simulink model "reference_frames_development"  (R2022a)
settings: Solver=VariableStepAuto  StartTime=0.0  StopTime=10.0  RelTol=1e-3
settings Model: Creator=samuel  LastModifiedBy=samuel

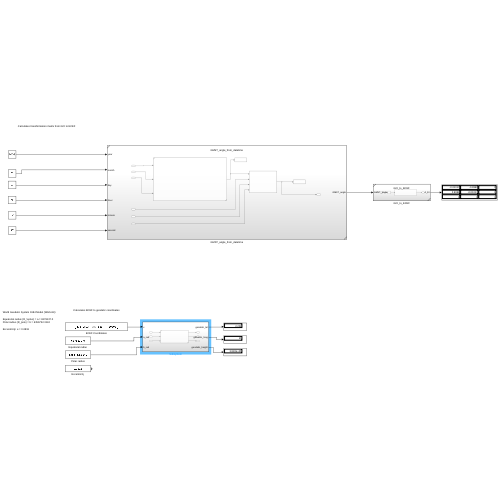
[thumbnail: Simulink's stored preview of the top-level diagram]
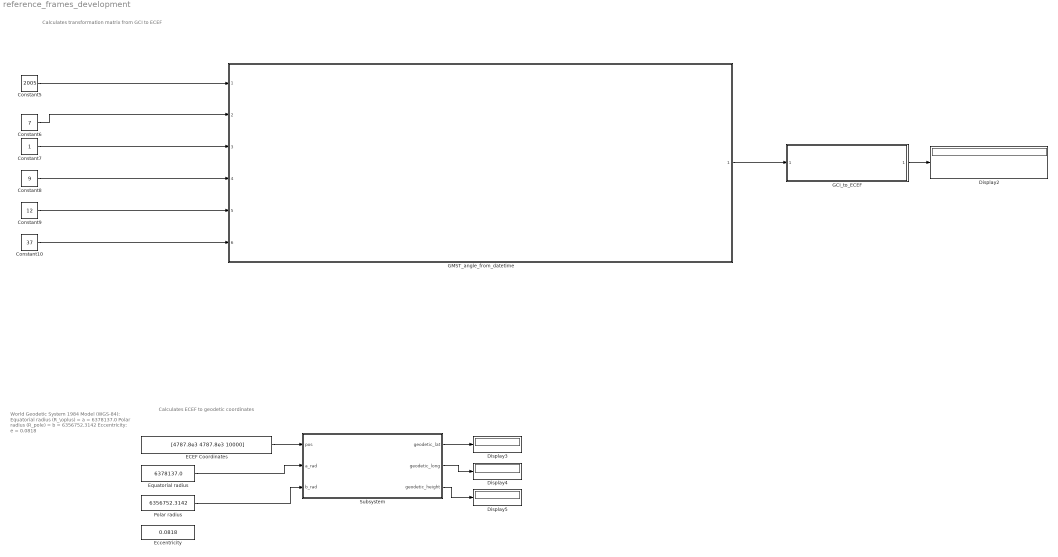
== system reference_frames_development ==
  note: Calculates transformation matrix from GCI to ECEF
  note: Calculates ECEF to geodetic coordinates
  note: World Geodetic System 1984 Model (WGS-84):
      |
      | Equatorial radius (R_\oplus) = a = 6378137.0
      | Polar radius (R_pole) = b = 6356752.3142
      |
      | Eccentricity: e = 0.0818
  Constant10 : Constant  Value=37
  Constant5 : Constant  Value=2005
  Constant6 : Constant  Value=7
  Constant7 : Constant
  Constant8 : Constant  Value=9
  Constant9 : Constant  Value=12
  Display{2..5} (4 alike) : Display
  ECEF Coordinates : Constant  Value=[4787.8e3 4787.8e3 10000]
  Eccentricity : Constant  Value=0.0818
  Equatorial radius : Constant  Value=6378137.0
  GCI_to_ECEF : Subsystem  ReferencedSubsystem=GCI_to_ECEF
  "GMST_angle_from_datetime " : Subsystem  ReferencedSubsystem=GMST_angle_from_datetime
  Polar radius : Constant  Value=6356752.3142
  Subsystem : Subsystem
  wires:
  Constant5/1 -> "GMST_angle_from_datetime "/1
  Constant6/1 -> "GMST_angle_from_datetime "/2
  Constant7/1 -> "GMST_angle_from_datetime "/3
  Constant8/1 -> "GMST_angle_from_datetime "/4
  Constant9/1 -> "GMST_angle_from_datetime "/5
  Constant10/1 -> "GMST_angle_from_datetime "/6
  "GMST_angle_from_datetime "/1 -> GCI_to_ECEF/1
  GCI_to_ECEF/1 -> Display2/1
  ECEF Coordinates/1 -> Subsystem/1(pos)
  Equatorial radius/1 -> Subsystem/2(a_rad)
  Polar radius/1 -> Subsystem/3(b_rad)
  Subsystem/1(geodetic_lat) -> Display3/1
  Subsystem/2(geodetic_long) -> Display4/1
  Subsystem/3(geodetic_height) -> Display5/1

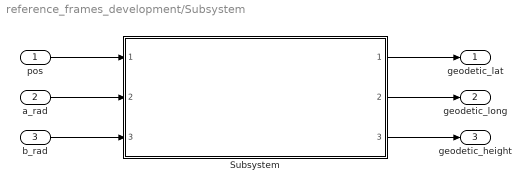
== system reference_frames_development/Subsystem ==
  pos : Inport
  a_rad : Inport  Port=2
  b_rad : Inport  Port=3
  Subsystem : Subsystem  ReferencedSubsystem=ECEF_coords_to_geodetic
  geodetic_lat : Outport
  geodetic_long : Outport  Port=2
  geodetic_height : Outport  Port=3
  wires:
  pos/1 -> Subsystem/1
  a_rad/1 -> Subsystem/2
  b_rad/1 -> Subsystem/3
  Subsystem/1 -> geodetic_lat/1
  Subsystem/2 -> geodetic_long/1
  Subsystem/3 -> geodetic_height/1
